simulink model "example_CondensingBoiler"  (R2016b)
settings: Solver=ode45  StartTime=0.0  StopTime=1*24*3600  MaxStep=1800  RelTol=1e-4  AbsTol=1e-5  EnableMultiTasking=on
undefined symbols (not defined in the file): path_carnot
libraries: carnot x6, simulink x2
settings Model: Creator=drhf  LastModifiedBy=drhf
settings DataIOCC: LimitDataPoints=on  SaveFormat=Array  SignalLoggingSaveFormat=ModelDataLogs
settings OptimizationCC: ExpressionDepthLimit=2147483647  LifeSpan=inf
settings DebuggingCC: UnderspecifiedInitializationDetection=Classic  MergeDetectMultiDrivingBlocksExec=none  SolverPrmCheckMsg=warning  FcnCallInpInsideContextMsg=warning  StateNameClashWarn=warning  SFUnexpectedBacktrackingDiag=warning  SFNoUnconditionalDefaultTransitionDiag=warning  SFExecutionAtInitializationDiag=none
settings HardwareCC: ProdBitPerPointer=32  ProdBitPerSizeT=32  ProdBitPerPtrDiffT=32  ProdLargestAtomicFloat=None  ProdIntDivRoundTo=Undefined  ProdEndianess=Unspecified  ProdWordSize=32  ProdHWDeviceType=32-bit Generic
settings ModelReferenceCC: PropagateSignalLabelsOutOfModel=off
settings GRTTargetCC: TargetLangStandard=C89/C90 (ANSI)  GeneratePreprocessorConditionals=Disable all  CombineOutputUpdateFcns=off  GRTInterface=on
settings ConfigComp: CovMetricSettings=dw  CovHtmlReporting=on  CovSaveCumulativeToWorkspaceVar=on  CovSaveSingleToWorkspaceVar=on  CovExternalEMLEnable=off

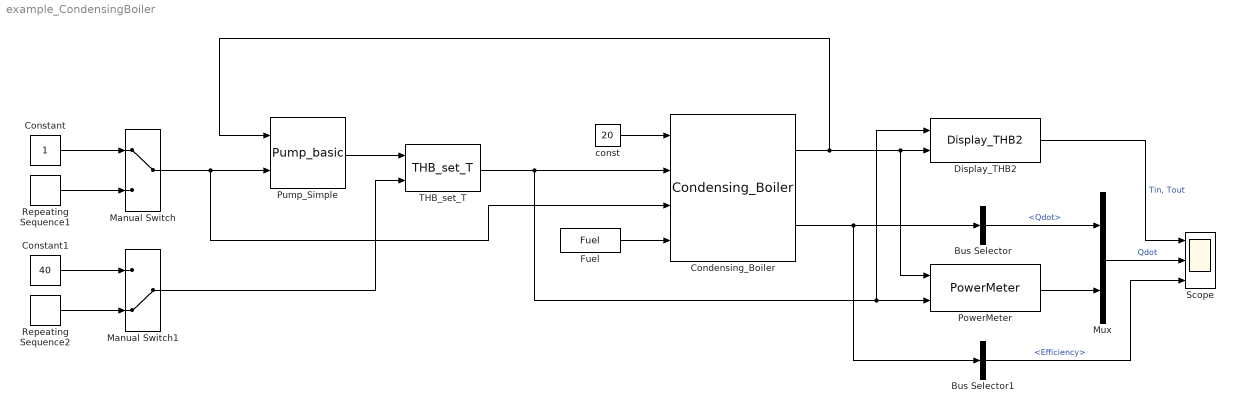
== system example_CondensingBoiler ==
  Bus Selector : BusSelector  OutputSignals=Qdot
  Bus Selector1 : BusSelector  OutputSignals=eco.Efficiency
  Condensing_Boiler : carnot/Source/Boiler/Condensing_Boiler  Tini=20  PathName=fullfile(path_carnot('libsl'), 'Source', 'Boiler', 'Condensing_Boiler', 'parameter_set')  FileName='CondensingBoiler_20kW.mat'  userPath=off  userParam=off  Pgas=20000  HeatLoss=2.5  Volume=0.0035  whichTforEfficiency=mean of inlet and outlet temperature  TableRelativePower=[0 0.1 1]  TableTemperatures=[10 50 90]  TableData=[1 1 1; 1.08 0.92 0.85; 1.06 0.9 0.83]  ElectricPower=[0 50 200]  relQdotMin=0.1  dplin=10  dpqua=100  nodes=3
  Constant : Constant
  Constant1 : Constant  Value=40
  Display_THB2 : carnot/Outputs/Display_THB2  t=on  m=off  p=off  id=off  mix=off  d=off
  Fuel : carnot/Source/Energy/Fuel  ft=1  t=20  ls=1  p=1e5  h_values=[5.14e7 5.69e7]  tc=45  price=1  mass=[0.33 0.67 0 0 0 0]
  Manual Switch : ManualSwitch
  Manual Switch1 : ManualSwitch  CurrentSetting=0
  Mux : Mux  Inputs=2
  PowerMeter : carnot/Control/PowerMeter
  Pump_Simple : carnot/Hydraulics/Pump_basic  mdotmax=2000/3600  fluid_id=Water  mix=0  mix2=0  mix3=0  p0=3e5  dia=0.0157  ID=No Pressure Drop  hgt=0
  Repeating Sequence1 : simulink/Sources/Repeating Sequence  rep_seq_t=[0 6 12]*3600  rep_seq_y=[0 1 0]
  Repeating Sequence2 : simulink/Sources/Repeating Sequence  rep_seq_t=[0 6 12]*3600  rep_seq_y=[20 70 20]
  Scope : Scope  NumInputPorts=3
  THB_set_T : carnot/Source/Simple/THB_set_T
  const : Constant  Value=20
  wires:
  const/1 -> Condensing_Boiler/1
  THB_set_T/1 -> PowerMeter/2, Display_THB2/1, Condensing_Boiler/2
  Fuel/1 -> Condensing_Boiler/4
  Condensing_Boiler/1 -> PowerMeter/1, Display_THB2/2, Pump_Simple/1
  Display_THB2/1 -> Scope/1  "Tin, Tout"
  Condensing_Boiler/2 -> Bus Selector/1, Bus Selector1/1
  Mux/1 -> Scope/2  "Qdot"
  PowerMeter/1 -> Mux/2
  Bus Selector/1 -> Mux/1  "<Qdot>"
  Pump_Simple/1 -> THB_set_T/1
  Manual Switch/1 -> Condensing_Boiler/3, Pump_Simple/2
  Constant/1 -> Manual Switch/1
  Repeating Sequence1/1 -> Manual Switch/2
  Constant1/1 -> Manual Switch1/1
  Repeating Sequence2/1 -> Manual Switch1/2
  Manual Switch1/1 -> THB_set_T/2
  Bus Selector1/1 -> Scope/3  "<Efficiency>"
